simulink model "SysTheoryNo3Model"  (R2023a)
settings: Solver=VariableStepAuto  StartTime=0.0  StopTime=sysTime  RelTol=1e-3
values from neighbouring files (symbols this model uses):
  disturbPower = 0    [SysTheoryNo3.m]
  disturbTime = 1    [SysTheoryNo3.m]
  noiseTime = 1    [SysTheoryNo3.m]
  sysA = double(subs(symA, paramArray, paramValues{paramChoise}))    [SysTheoryNo3.m]    (also in SysTheoryNo4.m)
  sysAnoise = double(subs(symA, paramArray, paramValuesNoise))    [SysTheoryNo3.m]    (also in SysTheoryNo4.m)
  sysB = double(subs(symB, paramArray, paramValues{paramChoise}))    [SysTheoryNo3.m]    (also in SysTheoryNo4.m)
  sysBnoise = double(subs(symB, paramArray, paramValuesNoise))    [SysTheoryNo3.m]    (also in SysTheoryNo4.m)
  sysC = [ ... (first row only)    [SysTheoryNo3.m]    (also in SysTheoryNo4.m)
  sysD = 0    [SysTheoryNo3.m]    (also in SysTheoryNo4.m)
  sysInit = [q1Init; q2Init; dq1Init; dq2Init]    [SysTheoryNo3.m]    (also in SysTheoryNo4.m)
  sysM = double(subs(symM, paramArray, paramValues{paramChoise}))    [SysTheoryNo3.m]
  sysVfast = - transpose(sysF)    [SysTheoryNo3.m]
  sysVkmnn = transpose(sysVkmnn)    [SysTheoryNo3.m]
  sysVslow = - transpose(sysF)    [SysTheoryNo3.m]
libraries: simulink x1
settings Model: Creator=utente  LastModifiedBy=utente

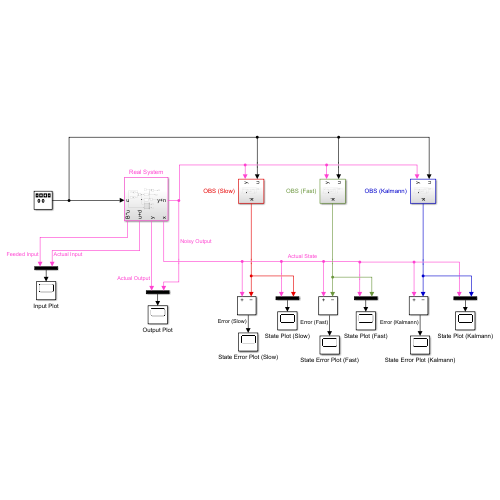
[thumbnail: Simulink's stored preview of the top-level diagram]
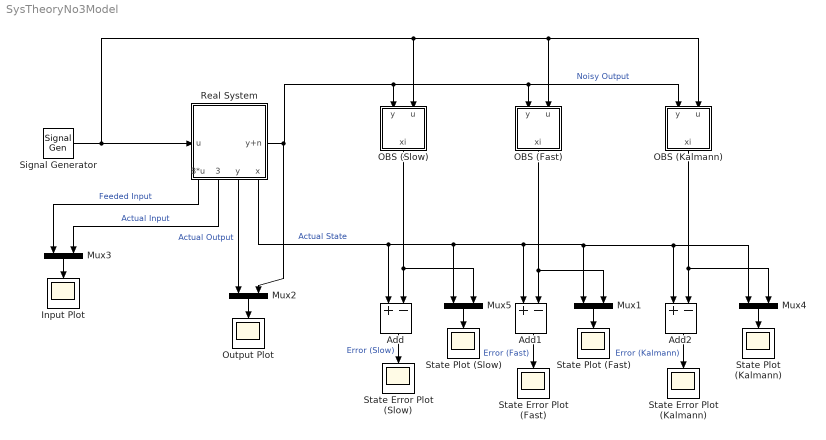
== system SysTheoryNo3Model ==
  Add : Sum  Inputs=+-
  Add1 : Sum  Inputs=+-
  Add2 : Sum  Inputs=+-
  Input Plot : Scope
  Mux{1..5} (5 alike) : Mux  Inputs=2
  OBS (Fast) : Subsystem
  OBS (Kalmann) : Subsystem
  OBS (Slow) : Subsystem
  Output Plot : Scope
  Real System : Subsystem
      settings: PortSchema="{\"entries\":[{\"content\":{\"sides\":[{\"content\":{\"connectorIds\":[\"In1\"]},\"type\":\"ConnectorPlacement.EquallySpacedRectSide\",\"uuid\":\"3f08ca9c-a9e9-4c14-ba34-4844dd77a68b\"},{\"content\":{\"connectorIds\":[\"Out1\"],\"side\":\"RIGHT\"},\"type\":\"ConnectorPlacement.EquallySpacedRectSide\",\"uuid\":\"bdc8f5f7-fa85-46de-82dd-bf8f95502a76\"},{\"content\":{\"side\":\"TOP\"},\"type\":\"ConnectorPlacement.EquallySpacedRectSide\",\"uuid\":\"be8b0dc5-8cbf-4fcd-8647-5527bbed652d\"},{\"content\":{\"connectorIds\":[\"Out2\",\"Out3\",\"Out4\",\"Out5\"],\"side\":\"BOTTOM\"},\"type\":\"ConnectorPlacement.EquallySpacedRectSide\",\"uuid\":\"310853c6-6c9e-4f78-8fe6-9cc81df5443e\"}]},\"type\":\"ConnectorPlacement.EquallySpacedConnector\",\"uuid\":\"8b960baf-3db8-48fd-9d4b-2c915c94d208\"}],\"packageUris\":[\"http://schema.mathworks.com/mf0/Connector/R2020b\"],\"version\":\"1.0\"}"
  Signal Generator : SignalGenerator  Frequency=2  Units=rad/sec
  State Error Plot (Fast) : Scope
  State Error Plot (Kalmann) : Scope
  State Error Plot (Slow) : Scope
  State Plot (Fast) : Scope
  State Plot (Kalmann) : Scope
  State Plot (Slow) : Scope
  wires:
  Signal Generator/1 -> OBS (Slow)/2(u), OBS (Kalmann)/2(u), OBS (Fast)/2(u), Real System/1(u)
  Add/1 -> State Error Plot (Slow)/1  "Error (Slow)"
  Real System/4(y) -> Mux2/1  "Actual Output"
  Mux2/1 -> Output Plot/1
  Real System/3(u+d) -> Mux3/2  "Actual Input"
  Mux3/1 -> Input Plot/1
  Real System/2(B*u) -> Mux3/1  "Feeded Input"
  Add1/1 -> State Error Plot (Fast)/1  "Error (Fast)"
  Add2/1 -> State Error Plot (Kalmann)/1  "Error (Kalmann)"
  Real System/1(y+n) -> OBS (Kalmann)/1(y), OBS (Fast)/1(y), OBS (Slow)/1(y), Mux2/2  "Noisy Output"
  OBS (Slow)/1(xi) -> Mux5/2, Add/2
  OBS (Fast)/1(xi) -> Mux1/2, Add1/2
  OBS (Kalmann)/1(xi) -> Mux4/2, Add2/2
  Real System/5(x) -> Mux4/1, Add2/1, Mux1/1, Add1/1, Mux5/1, Add/1  "Actual State"
  Mux5/1 -> State Plot (Slow)/1
  Mux1/1 -> State Plot (Fast)/1
  Mux4/1 -> State Plot (Kalmann)/1

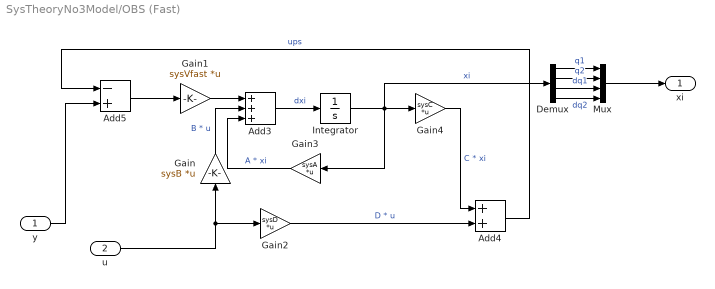
== system SysTheoryNo3Model/OBS (Fast) ==
  y : Inport
  u : Inport  Port=2
  Add3 : Sum  Inputs=+++
  Add4 : Sum
  Add5 : Sum  Inputs=-+
  Demux : Demux
  Gain : Gain  Gain=sysB  Multiplication=Matrix(K*u)
  Gain1 : Gain  Gain=sysVfast  Multiplication=Matrix(K*u)
  Gain2 : Gain  Gain=sysD  Multiplication=Matrix(K*u)
  Gain3 : Gain  Gain=sysA  Multiplication=Matrix(K*u)
  Gain4 : Gain  Gain=sysC  Multiplication=Matrix(K*u)
  Integrator : Integrator  InitialCondition=zeros(4, 1)
  Mux : Mux
  xi : Outport
  wires:
  Gain2/1 -> Add4/2  "D * u"
  Integrator/1 -> Demux/1, Gain3/1, Gain4/1  "xi"
  Gain/1 -> Add3/2  "B * u"
  Gain4/1 -> Add4/1  "C * xi"
  Gain3/1 -> Add3/3  "A * xi"
  u/1 -> Gain2/1, Gain/1
  Add3/1 -> Integrator/1  "dxi"
  Add5/1 -> Gain1/1
  Gain1/1 -> Add3/1
  Add4/1 -> Add5/1  "ups"
  y/1 -> Add5/2
  Demux/4 -> Mux/4  "dq2"
  Demux/3 -> Mux/3  "dq1"
  Demux/2 -> Mux/2  "q2"
  Demux/1 -> Mux/1  "q1"
  Mux/1 -> xi/1

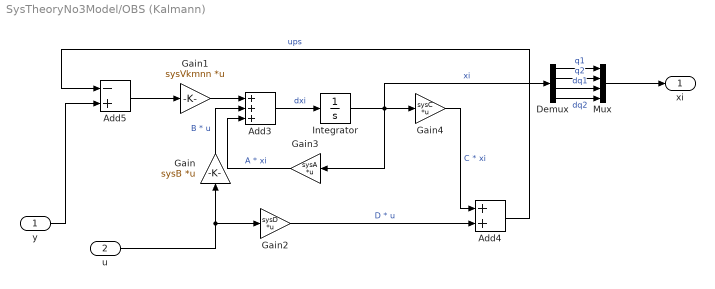
== system SysTheoryNo3Model/OBS (Kalmann) ==
  y : Inport
  u : Inport  Port=2
  Add3 : Sum  Inputs=+++
  Add4 : Sum
  Add5 : Sum  Inputs=-+
  Demux : Demux
  Gain : Gain  Gain=sysB  Multiplication=Matrix(K*u)
  Gain1 : Gain  Gain=sysVkmnn  Multiplication=Matrix(K*u)
  Gain2 : Gain  Gain=sysD  Multiplication=Matrix(K*u)
  Gain3 : Gain  Gain=sysA  Multiplication=Matrix(K*u)
  Gain4 : Gain  Gain=sysC  Multiplication=Matrix(K*u)
  Integrator : Integrator  InitialCondition=zeros(4, 1)
  Mux : Mux
  xi : Outport
  wires:
  Gain2/1 -> Add4/2  "D * u"
  Integrator/1 -> Demux/1, Gain3/1, Gain4/1  "xi"
  Gain/1 -> Add3/2  "B * u"
  Gain4/1 -> Add4/1  "C * xi"
  Gain3/1 -> Add3/3  "A * xi"
  u/1 -> Gain2/1, Gain/1
  Add3/1 -> Integrator/1  "dxi"
  Add5/1 -> Gain1/1
  Gain1/1 -> Add3/1
  Add4/1 -> Add5/1  "ups"
  y/1 -> Add5/2
  Demux/4 -> Mux/4  "dq2"
  Demux/3 -> Mux/3  "dq1"
  Demux/2 -> Mux/2  "q2"
  Demux/1 -> Mux/1  "q1"
  Mux/1 -> xi/1

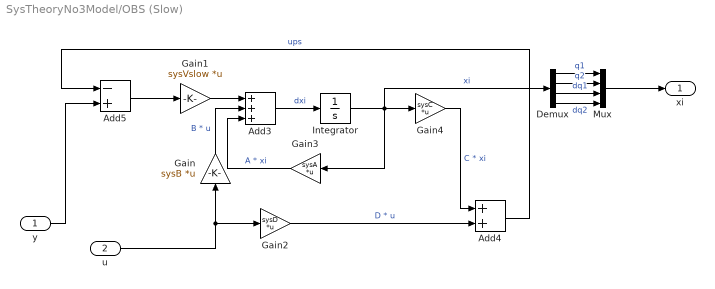
== system SysTheoryNo3Model/OBS (Slow) ==
  y : Inport
  u : Inport  Port=2
  Add3 : Sum  Inputs=+++
  Add4 : Sum
  Add5 : Sum  Inputs=-+
  Demux : Demux
  Gain : Gain  Gain=sysB  Multiplication=Matrix(K*u)
  Gain1 : Gain  Gain=sysVslow  Multiplication=Matrix(K*u)
  Gain2 : Gain  Gain=sysD  Multiplication=Matrix(K*u)
  Gain3 : Gain  Gain=sysA  Multiplication=Matrix(K*u)
  Gain4 : Gain  Gain=sysC  Multiplication=Matrix(K*u)
  Integrator : Integrator  InitialCondition=zeros(4, 1)
  Mux : Mux
  xi : Outport
  wires:
  Gain2/1 -> Add4/2  "D * u"
  Integrator/1 -> Demux/1, Gain3/1, Gain4/1  "xi"
  Gain/1 -> Add3/2  "B * u"
  Gain4/1 -> Add4/1  "C * xi"
  Gain3/1 -> Add3/3  "A * xi"
  u/1 -> Gain2/1, Gain/1
  Add3/1 -> Integrator/1  "dxi"
  Add5/1 -> Gain1/1
  Gain1/1 -> Add3/1
  Add4/1 -> Add5/1  "ups"
  y/1 -> Add5/2
  Demux/1 -> Mux/1  "q1"
  Demux/2 -> Mux/2  "q2"
  Demux/3 -> Mux/3  "dq1"
  Demux/4 -> Mux/4  "dq2"
  Mux/1 -> xi/1

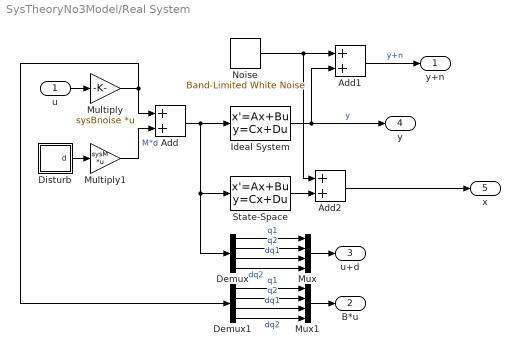
== system SysTheoryNo3Model/Real System ==
  u : Inport
  Add : Sum
  Add1 : Sum
  Add2 : Sum
  Demux : Demux
  Demux1 : Demux
  Disturb : Subsystem
  Ideal System : StateSpace  A=sysAnoise  B=eye(4)  C=sysC  D=sysD * zeros(1, 4)  InitialCondition=sysInit
  Multiply : Gain  Gain=sysBnoise  Multiplication=Matrix(K*u)
  Multiply1 : Gain  Gain=sysM  Multiplication=Matrix(K*u)
  Mux : Mux
  Mux1 : Mux
  Noise : simulink/Sources/Band-Limited White Noise  Cov=noisePower  Ts=noiseTime  seed=[23341]  VectorParams1D=off
  State-Space : StateSpace  A=sysAnoise  B=eye(4)  C=eye(4)  D=sysD * zeros(4, 4)  InitialCondition=sysInit
  y+n : Outport
  B*u : Outport  Port=2
  u+d : Outport  Port=3
  y : Outport  Port=4
  x : Outport  Port=5
  wires:
  Noise/1 -> Add2/1, Add1/1
  Ideal System/1 -> y/1, Add1/2  "y"
  Add1/1 -> y+n/1  "y+n"
  Disturb/1(d) -> Multiply1/1
  Multiply1/1 -> Add/2  "M*d"
  Add/1 -> State-Space/1, Demux/1, Ideal System/1
  Multiply/1 -> Demux1/1, Add/1
  u/1 -> Multiply/1
  Demux1/1 -> Mux1/1  "q1"
  Demux1/3 -> Mux1/3  "dq1"
  Demux1/4 -> Mux1/4  "dq2"
  Demux1/2 -> Mux1/2  "q2"
  Mux1/1 -> B*u/1
  Mux/1 -> u+d/1
  Demux/1 -> Mux/1  "q1"
  Demux/2 -> Mux/2  "q2"
  Demux/3 -> Mux/3  "dq1"
  Demux/4 -> Mux/4  "dq2"
  State-Space/1 -> Add2/2
  Add2/1 -> x/1

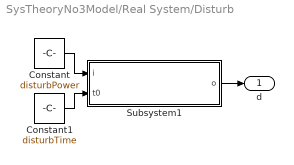
== system SysTheoryNo3Model/Real System/Disturb ==
  Constant : Constant  Value=disturbPower
  Constant1 : Constant  Value=disturbTime
  Subsystem1 : Subsystem
  d : Outport
  wires:
  Constant1/1 -> Subsystem1/2(t0)
  Subsystem1/1(o) -> d/1
  Constant/1 -> Subsystem1/1(i)

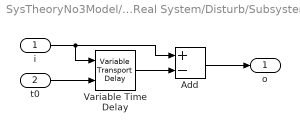
== system SysTheoryNo3Model/Real System/Disturb/Subsystem1 ==
  i : Inport
  t0 : Inport  Port=2
  Add : Sum  Inputs=+-
  Variable Time Delay : VariableTransportDelay  MaximumDelay=10
  o : Outport
  wires:
  i/1 -> Add/1, Variable Time Delay/1
  Add/1 -> o/1
  t0/1 -> Variable Time Delay/2
  Variable Time Delay/1 -> Add/2
